simulink model "Brazo"  (R2017a)
settings: Solver=VariableStepAuto  StartTime=0.0  StopTime=10.0  RelTol=1e-3
undefined symbols (not defined in the file): Brazo_Piezas
libraries: mblibv1 x10
settings Model: Creator=LuisFernando  LastModifiedBy=LuisFernando
settings SimMechanicsCC: VisOnUpdateDiagram=on  VisDuringSimulation=on

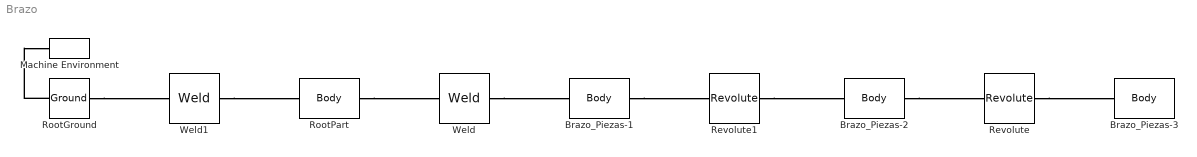
== system Brazo ==
  Brazo_Piezas-1 : mblibv1/Bodies/Body  LConnTagsString=CS2  RConnTagsString=CS3  UpdateFromCAD=on  PMImportedID=Brazo_Piezas-1  DialogClass=MechanicalBodyBlock  Mass=0.000948939  MassUnits=kg  InertiaUnits=kg*m^2  Inertia=[7.65593e-08,-8.75454e-08,0;-8.75454e-08,1.07768e-07,0;0,0,1.80373e-07]  Shape=Cylinder  ShapeDims=[1 1]  ShapeUnits=m  ShapeUse=false  Density=1  DensityUnits=kg/m^3  DensityUse=false  GraphicsMode=GFXFILE  GraphicsFileName=Brazo - Brazo_Piezas-1.STL  BodyColorSelMode=COLORPALETTE  BodyColor=[0.792157;0.819608;0.933333]  AttachedToCS=CS1  CG=Right$CG$[0.017555 0.0266927 0.0233856]$WORLD$WORLD$m$[1 0 0;0 1 0;0 0 1]$3x3 Transform$rad$WORLD$false$Brazo_Piezas-1::CG(AUTOGEN)  WorkingFrames=Right$CS1$[-0.0236944 0.0122459 0.0208856]$WORLD$WORLD$m$[1 0 0;0 1 0;0 0 1]$3x3 Transform$rad$WORLD$false$Brazo_Piezas-1::CS1(AUTOGEN)#Left$CS2$[0.017555 0.0266927 0.0233856]$WORLD$WORLD$m$[1 0 0;0 1 0;0 0 1]$3x3 Transform$rad$WORLD$true$Brazo/RootPart:-:Brazo_Piezas-1::Brazo_Piezas-1(AUTOGEN)#Right$CS3$[0.00030557 0.0122459 0.0258856]$WORLD$WORLD$m$[1 0 0;0 1 0;0 0 1]$3x3 Transform$rad$WORLD$true$Brazo_Piezas-1:-:Brazo_Piezas-2::Brazo_Piezas-1(AUTOGEN)  CGPos=[0.017555 0.0266927 0.0233856]  CGRot=[1 0 0;0 1 0;0 0 1]  CS0Pos=[]  CS0Rot=[]  CS1Pos=[-0.0236944 0.0122459 0.0208856]  CS1Rot=[1 0 0;0 1 0;0 0 1]  CS2Pos=[0.017555 0.0266927 0.0233856]  CS2Rot=[1 0 0;0 1 0;0 0 1]  CS3Pos=[0.00030557 0.0122459 0.0258856]  CS3Rot=[1 0 0;0 1 0;0 0 1]  CS4Pos=[]  CS4Rot=[]  CS5Pos=[]  CS5Rot=[]  CS6Pos=[]  CS6Rot=[]  CS7Pos=[]  CS7Rot=[]  CS8Pos=[]  CS8Rot=[]  CS9Pos=[]  CS9Rot=[]  CS10Pos=[]  CS10Rot=[]  CS11Pos=[]  CS11Rot=[]  CS12Pos=[]  CS12Rot=[]  CS13Pos=[]  CS13Rot=[]  CS14Pos=[]  CS14Rot=[]  CS15Pos=[]  CS15Rot=[]  CS16Pos=[]  CS16Rot=[]  CS17Pos=[]  CS17Rot=[]  CS18Pos=[]  CS18Rot=[]  CS19Pos=[]  CS19Rot=[]  CS20Pos=[]  CS20Rot=[]
      settings: SourceProductName=Simscape Multibody  SourceProductBaseCode=MS
  Brazo_Piezas-2 : mblibv1/Bodies/Body  LConnTagsString=CS3  RConnTagsString=CS2  UpdateFromCAD=on  PMImportedID=Brazo_Piezas-2  DialogClass=MechanicalBodyBlock  Mass=0.000888939  MassUnits=kg  InertiaUnits=kg*m^2  Inertia=[3.04145e-09,-1.09497e-09,0;-1.09497e-09,1.49207e-07,0;0,0,1.48545e-07]  Shape=Cylinder  ShapeDims=[1 1]  ShapeUnits=m  ShapeUse=false  Density=1  DensityUnits=kg/m^3  DensityUse=false  GraphicsMode=GFXFILE  GraphicsFileName=Brazo - Brazo_Piezas-2.STL  BodyColorSelMode=COLORPALETTE  BodyColor=[0.792157;0.819608;0.933333]  AttachedToCS=CS1  CG=Right$CG$[-0.0128537 0.0286116 0.0283856]$WORLD$WORLD$m$[0.620775 0.783989 0;-0.783989 0.620775 0;0 0 1]$3x3 Transform$rad$WORLD$false$Brazo_Piezas-2::CG(AUTOGEN)  WorkingFrames=Right$CS1$[-0.0586612 0.0401721 0.0258856]$WORLD$WORLD$m$[0.620775 0.783989 0;-0.783989 0.620775 0;0 0 1]$3x3 Transform$rad$WORLD$false$Brazo_Piezas-2::CS1(AUTOGEN)#Right$CS2$[0.00030557 0.0122459 0.0308856]$WORLD$WORLD$m$[1 0 0;0 1 0;0 0 1]$3x3 Transform$rad$WORLD$true$Brazo_Piezas-2:-:Brazo_Piezas-3::Brazo_Piezas-2(AUTOGEN)#Left$CS3$[0.00030557 0.0122459 0.0258856]$WORLD$WORLD$m$[1 0 0;0 1 0;0 0 1]$3x3 Transform$rad$WORLD$true$Brazo_Piezas-1:-:Brazo_Piezas-2::Brazo_Piezas-2(AUTOGEN)  CGPos=[-0.0128537 0.0286116 0.0283856]  CGRot=[0.620775 0.783989 0;-0.783989 0.620775 0;0 0 1]  CS0Pos=[]  CS0Rot=[]  CS1Pos=[-0.0586612 0.0401721 0.0258856]  CS1Rot=[0.620775 0.783989 0;-0.783989 0.620775 0;0 0 1]  CS2Pos=[0.00030557 0.0122459 0.0308856]  CS2Rot=[1 0 0;0 1 0;0 0 1]  CS3Pos=[0.00030557 0.0122459 0.0258856]  CS3Rot=[1 0 0;0 1 0;0 0 1]  CS4Pos=[]  CS4Rot=[]  CS5Pos=[]  CS5Rot=[]  CS6Pos=[]  CS6Rot=[]  CS7Pos=[]  CS7Rot=[]  CS8Pos=[]  CS8Rot=[]  CS9Pos=[]  CS9Rot=[]  CS10Pos=[]  CS10Rot=[]  CS11Pos=[]  CS11Rot=[]  CS12Pos=[]  CS12Rot=[]  CS13Pos=[]  CS13Rot=[]  CS14Pos=[]  CS14Rot=[]  CS15Pos=[]  CS15Rot=[]  CS16Pos=[]  CS16Rot=[]  CS17Pos=[]  CS17Rot=[]  CS18Pos=[]  CS18Rot=[]  CS19Pos=[]  CS19Rot=[]  CS20Pos=[]  CS20Rot=[]
      settings: SourceProductName=Simscape Multibody  SourceProductBaseCode=MS
  Brazo_Piezas-3 : mblibv1/Bodies/Body  LConnTagsString=CS2  UpdateFromCAD=on  PMImportedID=Brazo_Piezas-3  DialogClass=MechanicalBodyBlock  Mass=1.38929e-05  MassUnits=kg  InertiaUnits=kg*m^2  Inertia=[1.1731e-10,0,0;0,1.1731e-10,0;0,0,3.0719e-12]  Shape=Cylinder  ShapeDims=[1 1]  ShapeUnits=m  ShapeUse=false  Density=1  DensityUnits=kg/m^3  DensityUse=false  GraphicsMode=GFXFILE  GraphicsFileName=Brazo - Brazo_Piezas-3.STL  BodyColorSelMode=COLORPALETTE  BodyColor=[0.792157;0.819608;0.933333]  AttachedToCS=CS1  CG=Right$CG$[0.00030557 0.0122459 0.0258856]$WORLD$WORLD$m$[0.781211 -0.624268 0;0.624268 0.781211 0;0 0 1]$3x3 Transform$rad$WORLD$false$Brazo_Piezas-3::CG(AUTOGEN)  WorkingFrames=Right$CS1$[0.00525644 -0.0203806 0.0258856]$WORLD$WORLD$m$[0.781211 -0.624268 0;0.624268 0.781211 0;0 0 1]$3x3 Transform$rad$WORLD$false$Brazo_Piezas-3::CS1(AUTOGEN)#Left$CS2$[0.00030557 0.0122459 0.0308856]$WORLD$WORLD$m$[1 0 0;0 1 0;0 0 1]$3x3 Transform$rad$WORLD$true$Brazo_Piezas-2:-:Brazo_Piezas-3::Brazo_Piezas-3(AUTOGEN)  CGPos=[0.00030557 0.0122459 0.0258856]  CGRot=[0.781211 -0.624268 0;0.624268 0.781211 0;0 0 1]  CS0Pos=[]  CS0Rot=[]  CS1Pos=[0.00525644 -0.0203806 0.0258856]  CS1Rot=[0.781211 -0.624268 0;0.624268 0.781211 0;0 0 1]  CS2Pos=[0.00030557 0.0122459 0.0308856]  CS2Rot=[1 0 0;0 1 0;0 0 1]  CS3Pos=[]  CS3Rot=[]  CS4Pos=[]  CS4Rot=[]  CS5Pos=[]  CS5Rot=[]  CS6Pos=[]  CS6Rot=[]  CS7Pos=[]  CS7Rot=[]  CS8Pos=[]  CS8Rot=[]  CS9Pos=[]  CS9Rot=[]  CS10Pos=[]  CS10Rot=[]  CS11Pos=[]  CS11Rot=[]  CS12Pos=[]  CS12Rot=[]  CS13Pos=[]  CS13Rot=[]  CS14Pos=[]  CS14Rot=[]  CS15Pos=[]  CS15Rot=[]  CS16Pos=[]  CS16Rot=[]  CS17Pos=[]  CS17Rot=[]  CS18Pos=[]  CS18Rot=[]  CS19Pos=[]  CS19Rot=[]  CS20Pos=[]  CS20Rot=[]
      settings: SourceProductName=Simscape Multibody  SourceProductBaseCode=MS
  Machine Environment : mblibv1/Bodies/Machine Environment  PortType=env  PhysicalDomain=Mechanical  DialogTemplateClass=MECH.MachineEnvironment  SyncWhenCopied=off  Gravity=[0 -9.81 0]  GravityUnits=m/s^2  GravityAsSignal=off  Dimensionality=Auto-detect  AnalysisType=Forward dynamics  LinearAssemblyTolerance=1e-3  LinearAssemblyToleranceUnits=m  AngularAssemblyTolerance=1e-3  AngularAssemblyToleranceUnits=rad  ConstraintSolverType=Stabilizing  ConstraintRelTolerance=1e-4  ConstraintAbsTolerance=1e-4  UseRobustSingularityHandling=off  RedundancyAnalysisToleranceType=Automatically select tolerance  RedundancyAnalysisTolerance=1e-14  StatePerturbationType=Fixed  PerturbationSize=1e-5  VisualizeMachine=on  BodyVisualizationType=Use model default body geometries  BodyColorSelMode=Use model default  DefaultBodyColor=[1 0 0]
      settings: SourceProductName=Simscape Multibody  SourceProductBaseCode=MS
  Revolute : mblibv1/Joints/Revolute  LConnTagsString=__newl0  RConnTagsString=__newr0  UpdateFromCAD=on  PMImportedID=Brazo_Piezas-2:-:Brazo_Piezas-3  NumSAPorts=0  CutJoint=off  MarkAsCut=off  Primitives=prismatic  PrimitiveProps=R1$WORLD$[0,0,1]$revolute  DialogClass=JointBlock  R1Axis=[0,0,1]
      settings: SourceProductName=Simscape Multibody  SourceProductBaseCode=MS
  Revolute1 : mblibv1/Joints/Revolute  LConnTagsString=__newl0  RConnTagsString=__newr0  UpdateFromCAD=on  PMImportedID=Brazo_Piezas-1:-:Brazo_Piezas-2  NumSAPorts=0  CutJoint=off  MarkAsCut=off  Primitives=prismatic  PrimitiveProps=R1$WORLD$[0,0,1]$revolute  DialogClass=JointBlock  R1Axis=[0,0,1]
      settings: SourceProductName=Simscape Multibody  SourceProductBaseCode=MS
  RootGround : mblibv1/Bodies/Ground  UpdateFromCAD=on  PMImportedID=RootGround  LeftPortType=env  RightPortType=workingframe  PhysicalDomain=Mechanical  DialogClass=GroundBlock  CoordPosition=[0.00282796,0.0275055,0.0258046]  CoordPositionUnits=m  StateVectorMgrId=0  MachineId=[1 0]  ShowEnvPort=on  ParameterChecksum=[251060669, 366471734, 2618027187, 50697566]  TopologyChecksum=[3221416587, 2481637375, 25109446, 3942316502]
      settings: SourceProductName=Simscape Multibody  SourceProductBaseCode=MS
  RootPart : mblibv1/Bodies/Body  LConnTagsString=CS3  RConnTagsString=CS2  UpdateFromCAD=on  PMImportedID=Brazo/RootPart  DialogClass=MechanicalBodyBlock  Mass=0  MassUnits=kg  InertiaUnits=kg*m^2  Inertia=[0,0,0;0,0,0;0,0,0]  Shape=Cylinder  ShapeDims=[1 1]  ShapeUnits=m  ShapeUse=false  Density=1  DensityUnits=kg/m^3  DensityUse=false  GraphicsMode=MACHINE_DEFAULT  BodyColorSelMode=MACHINE_DEFAULT  BodyColor=[1;0;0]  AttachedToCS=CS1  CG=Right$CG$[0.00282796 0.0275055 0.0258046]$WORLD$WORLD$m$[1 0 0;0 1 0;0 0 1]$3x3 Transform$rad$WORLD$false$Brazo/RootPart::CG(AUTOGEN)  WorkingFrames=Right$CS1$[0 0 0]$WORLD$WORLD$m$[1 0 0;0 1 0;0 0 1]$3x3 Transform$rad$WORLD$false$Brazo/RootPart::CS1(AUTOGEN)#Right$CS2$[0.017555 0.0266927 0.0233856]$WORLD$WORLD$m$[1 0 0;0 1 0;0 0 1]$3x3 Transform$rad$WORLD$true$Brazo/RootPart:-:Brazo_Piezas-1::Brazo/RootPart(AUTOGEN)#Left$CS3$[0.00282796 0.0275055 0.0258046]$WORLD$WORLD$m$[1 0 0;0 1 0;0 0 1]$3x3 Transform$rad$WORLD$true$Brazo/RootPart:-:RootGround::Brazo/RootPart(AUTOGEN)  CGPos=[0.00282796 0.0275055 0.0258046]  CGRot=[1 0 0;0 1 0;0 0 1]  CS0Pos=[]  CS0Rot=[]  CS1Pos=[0 0 0]  CS1Rot=[1 0 0;0 1 0;0 0 1]  CS2Pos=[0.017555 0.0266927 0.0233856]  CS2Rot=[1 0 0;0 1 0;0 0 1]  CS3Pos=[0.00282796 0.0275055 0.0258046]  CS3Rot=[1 0 0;0 1 0;0 0 1]  CS4Pos=[]  CS4Rot=[]  CS5Pos=[]  CS5Rot=[]  CS6Pos=[]  CS6Rot=[]  CS7Pos=[]  CS7Rot=[]  CS8Pos=[]  CS8Rot=[]  CS9Pos=[]  CS9Rot=[]  CS10Pos=[]  CS10Rot=[]  CS11Pos=[]  CS11Rot=[]  CS12Pos=[]  CS12Rot=[]  CS13Pos=[]  CS13Rot=[]  CS14Pos=[]  CS14Rot=[]  CS15Pos=[]  CS15Rot=[]  CS16Pos=[]  CS16Rot=[]  CS17Pos=[]  CS17Rot=[]  CS18Pos=[]  CS18Rot=[]  CS19Pos=[]  CS19Rot=[]  CS20Pos=[]  CS20Rot=[]
      settings: SourceProductName=Simscape Multibody  SourceProductBaseCode=MS
  Weld : mblibv1/Joints/Weld  LConnTagsString=__newl0  RConnTagsString=__newr0  UpdateFromCAD=on  PMImportedID=Brazo/RootPart:-:Brazo_Piezas-1  NumSAPorts=0  CutJoint=off  MarkAsCut=off  Primitives=weld  PrimitiveProps=W$WORLD$[0.57735,0.57735,0.57735]$weld  DialogClass=JointBlock  WAxis=[0.57735,0.57735,0.57735]
      settings: SourceProductName=Simscape Multibody  SourceProductBaseCode=MS
  Weld1 : mblibv1/Joints/Weld  LConnTagsString=__newl0  RConnTagsString=__newr0  UpdateFromCAD=on  PMImportedID=Brazo/RootPart:-:RootGround  NumSAPorts=0  CutJoint=off  MarkAsCut=off  Primitives=weld  PrimitiveProps=W$WORLD$[0.57735,0.57735,0.57735]$weld  DialogClass=JointBlock  WAxis=[0.57735,0.57735,0.57735]
      settings: SourceProductName=Simscape Multibody  SourceProductBaseCode=MS
  connections:
  RootPart/RConn1 -- Weld/LConn1
  Weld/RConn1 -- Brazo_Piezas-1/LConn1
  Brazo_Piezas-2/RConn1 -- Revolute/LConn1
  Revolute/RConn1 -- Brazo_Piezas-3/LConn1
  Brazo_Piezas-1/RConn1 -- Revolute1/LConn1
  Revolute1/RConn1 -- Brazo_Piezas-2/LConn1
  RootGround/RConn1 -- Weld1/LConn1
  Weld1/RConn1 -- RootPart/LConn1
  RootGround/LConn1 -- Machine Environment/RConn1
